simulink model "a1"  (R2012b)
settings: Solver=ode45  StartTime=0.0  StopTime=10.0  RelTol=1e-3
libraries: simulink x1
settings Model: Creator=ZhouHaoyu  LastModifiedBy=ZhouHaoyu

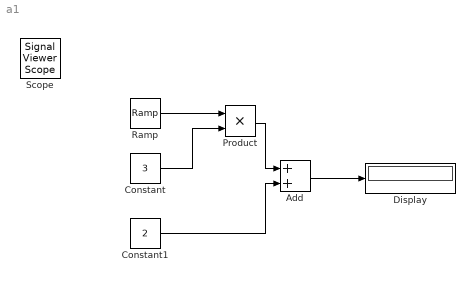
== system a1 ==
  Add : Sum
  Constant : Constant  Value=3
  Constant1 : Constant  Value=2
  Display : Display
  Product : Product  RndMeth=Zero
  Ramp : simulink/Sources/Ramp  slope=1  start=0  X0=0
  Scope : SignalViewerScope  IOType=viewer  RefreshTime=0.035000
  wires:
  Constant/1 -> Product/2
  Ramp/1 -> Product/1
  Product/1 -> Add/1
  Constant1/1 -> Add/2
  Add/1 -> Display/1
